simulink model "motor_bldc"  (R2022b)
settings: Solver=VariableStepAuto  StartTime=0.0  StopTime=0.2  RelTol=1e-3
values from neighbouring files (symbols this model uses):
  Bm = Bms(i)    [sim_motor.m]    (also in var_motor.m = 0.0005)
  fm = PSIs(i)    [sim_motor.m]    (also in var_motor.m = 0.15)
  J = Js(i)    [sim_motor.m]    (also in var_motor.m = 0.00025)
  Lmb = Lss - Lls    (= 0.0045)    [sim_motor.m]    (also in var_motor.m)
  Lss = 5e-3    (= 0.005)    [sim_motor.m]    (also in var_motor.m)
  P = 4    [sim_motor.m]    (also in var_motor.m)
  rs = RSs(i)    [sim_motor.m]    (also in var_motor.m = 1)
  TL = 0    [sim_motor.m]    (also in var_motor.m = 0.3)
  uM = 50    [sim_motor.m]    (also in var_motor.m)
settings Model: Creator=andre  LastModifiedBy=andre

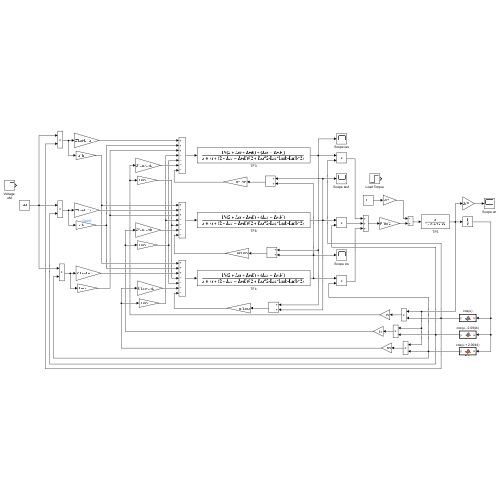
[thumbnail: Simulink's stored preview of the top-level diagram]
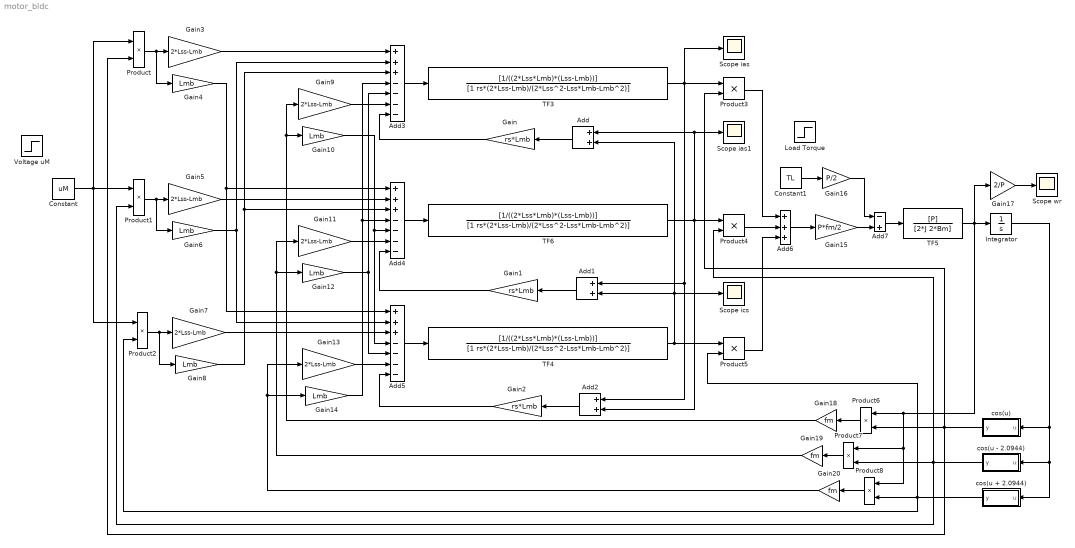
== system motor_bldc ==
  Add : Sum
  Add1 : Sum
  Add2 : Sum
  Add3 : Sum  Inputs=+++----
  Add4 : Sum  Inputs=+++----
  Add5 : Sum  Inputs=+++----
  Add6 : Sum  Inputs=+++
  Add7 : Sum  Inputs=-+
  Constant : Constant  Value=uM
  Constant1 : Constant  Value=TL
  Gain : Gain  Gain=rs*Lmb
  Gain1 : Gain  Gain=rs*Lmb
  Gain{4,6,8,10,12,14} (6 alike) : Gain  Gain=Lmb
  Gain{3,5,7,9,11,13} (6 alike) : Gain  Gain=2*Lss-Lmb
  Gain15 : Gain  Gain=P*fm/2
  Gain16 : Gain  Gain=P/2
  Gain17 : Gain  Gain=2/P
  Gain18 : Gain  Gain=fm
  Gain19 : Gain  Gain=fm
  Gain2 : Gain  Gain=rs*Lmb
  Gain20 : Gain  Gain=fm
  Integrator : Integrator
  Load Torque : Step  After=TL  SampleTime=0
  Product{,1..8} (9 alike) : Product
  Scope ias : Scope
  Scope ias1 : Scope
  Scope ics : Scope
  Scope wr : Scope
  TF3 : TransferFcn  Numerator=[1/((2*Lss*Lmb)*(Lss-Lmb))]  Denominator=[1 rs*(2*Lss-Lmb)/(2*Lss^2-Lss*Lmb-Lmb^2)]
  TF4 : TransferFcn  Numerator=[1/((2*Lss*Lmb)*(Lss-Lmb))]  Denominator=[1 rs*(2*Lss-Lmb)/(2*Lss^2-Lss*Lmb-Lmb^2)]
  TF5 : TransferFcn  Numerator=[P]  Denominator=[2*J 2*Bm]
  TF6 : TransferFcn  Numerator=[1/((2*Lss*Lmb)*(Lss-Lmb))]  Denominator=[1 rs*(2*Lss-Lmb)/(2*Lss^2-Lss*Lmb-Lmb^2)]
  Voltage uM : Step  After=uM  SampleTime=0
  cos(u + 2.0944) : MATLAB Function  TreatAsAtomicUnit=on
  cos(u - 2.0944) : MATLAB Function  TreatAsAtomicUnit=on
  cos(u) : MATLAB Function  TreatAsAtomicUnit=on
  wires:
  Add/1 -> Gain/1
  Add1/1 -> Gain1/1
  Add2/1 -> Gain2/1
  Add3/1 -> TF3/1
  Add4/1 -> TF6/1
  Add5/1 -> TF4/1
  Gain1/1 -> Add4/7
  Gain/1 -> Add3/7
  Gain2/1 -> Add5/7
  Product/1 -> Gain4/1, Gain3/1
  Gain3/1 -> Add3/1
  Product1/1 -> Gain6/1, Gain5/1
  Product2/1 -> Gain8/1, Gain7/1
  Constant/1 -> Product2/1, Product/1, Product1/1
  Gain9/1 -> Add3/6
  Gain11/1 -> Add4/6
  Gain13/1 -> Add5/6
  Gain5/1 -> Add4/2
  Gain4/1 -> Add5/1, Add4/1
  Gain7/1 -> Add5/3
  Gain6/1 -> Add3/2, Add5/2
  Gain12/1 -> Add3/5, Add5/5
  Gain10/1 -> Add5/4, Add4/5
  Gain14/1 -> Add3/4, Add4/4
  Gain8/1 -> Add3/3, Add4/3
  TF3/1 -> Add2/1, Add1/1, Product3/1, Scope ias/1
  TF6/1 -> Add/1, Scope ias1/1, Add2/2, Product4/1
  TF4/1 -> Add/2, Scope ics/1, Add1/2, Product5/1
  Product3/1 -> Add6/1
  Product4/1 -> Add6/2
  Product5/1 -> Add6/3
  Add6/1 -> Gain15/1
  Gain15/1 -> Add7/2
  Gain16/1 -> Add7/1
  Add7/1 -> TF5/1
  Gain17/1 -> Scope wr/1
  TF5/1 -> Product6/1, Product8/1, Product7/1, Integrator/1, Gain17/1
  Integrator/1 -> cos(u + 2.0944)/1(u), cos(u - 2.0944)/1(u), cos(u)/1(u)
  cos(u)/1(y) -> Product3/2, Product/2, Product6/2
  cos(u + 2.0944)/1(y) -> Product5/2, Product2/2, Product8/2
  cos(u - 2.0944)/1(y) -> Product4/2, Product1/2, Product7/2
  Product6/1 -> Gain18/1
  Product7/1 -> Gain19/1
  Product8/1 -> Gain20/1
  Gain18/1 -> Gain9/1, Gain10/1
  Gain19/1 -> Gain12/1, Gain11/1
  Gain20/1 -> Gain14/1, Gain13/1
  Constant1/1 -> Gain16/1

== matlab function motor_bldc/cos(u) ==
  data: u input; y output
function y = fcn(u)

y = cos(u);

== matlab function motor_bldc/cos(u + 2.0944) ==
  data: u input; y output
function y = fcn(u)

y = cos(u+2.0944);

== matlab function motor_bldc/cos(u - 2.0944) ==
  data: u input; y output
function y = fcn(u)

y = cos(u-2.0944);
